simulink model "ROEdamico2RTN"  (R2023a)
settings: Solver=ode4  StartTime=0.0  StopTime=10.0  FixedStep=dt  RelTol=1e-3
settings Model: Creator=ndelurgio  LastModifiedBy=ndelurgio

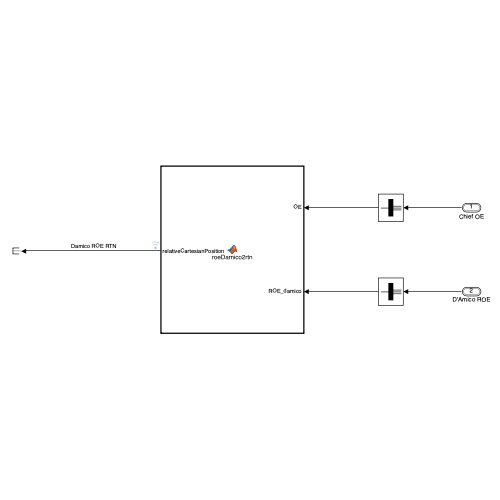
[thumbnail: Simulink's stored preview of the top-level diagram]
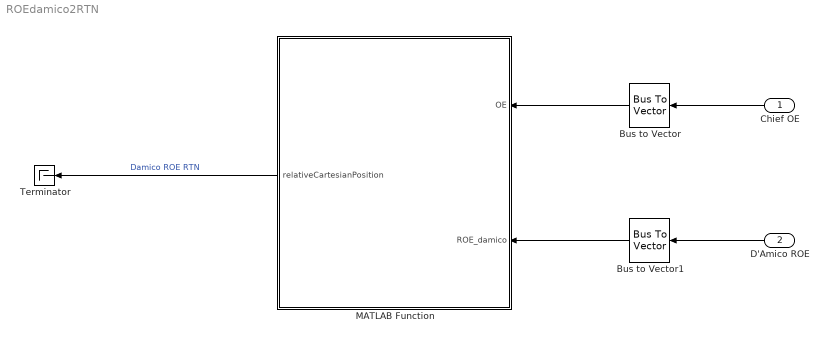
== system ROEdamico2RTN ==
  Chief OE : Inport  OutDataTypeStr=Bus: osculatingOrbitElements
  D'Amico ROE : Inport  Port=2  OutDataTypeStr=Bus: damicoROE
  Bus to Vector : BusToVector
  Bus to Vector1 : BusToVector
  MATLAB Function : MATLAB Function  TreatAsAtomicUnit=on
  Terminator : Terminator
  wires:
  Chief OE/1 -> Bus to Vector/1
  D'Amico ROE/1 -> Bus to Vector1/1
  Bus to Vector/1 -> MATLAB Function/1(OE)
  Bus to Vector1/1 -> MATLAB Function/2(ROE_damico)
  MATLAB Function/1(relativeCartesianPosition) -> Terminator/1  "Damico ROE RTN"

== matlab function ROEdamico2RTN/MATLAB Function ==
  data: OE input; ROE_damico input; relativeCartesianPosition output
function relativeCartesianPosition = roeDamico2rtn(OE,ROE_damico)
relativeCartesianPosition = roeDamico2rtn(ROE_damico,OE);
end
